simulink model "QCar2_Physical"  (R2025b)
settings: Solver=ode1  StartTime=0.0  StopTime=inf  FixedStep=Controller_Sample_Time  RelTol=1e-3  EnableMultiTasking=on
PreLoadFcn:
  | QCarSetup
values from neighbouring files (symbols this model uses):
  Audio_Sample_Time = 0.3    [QCarSetup.m]
  CSI_Sample_Time = 1/60    (= 0.0166666666667)    [QCarSetup.m]
  ImageDisplay_Sample_Time = 120*Controller_Sample_Time    (= 0.1)    [QCarSetup.m]
  LiDAR_Sample_Time = CSI_Sample_Time*3    (= 0.05)    [QCarSetup.m]
  NN_Sample_Time = RealSense_Sample_Time*1    (= 0.0333333333333)    [QCarSetup.m]
  RealSense_Sample_Time = CSI_Sample_Time*2    (= 0.0333333333333)    [QCarSetup.m]
undefined symbols (not defined in the file or in its folder): Cobra_Start, DiscIntNeverNeededParam, engine, gcbh, height, HIL, honk, Joystick_Sample_Time, JPEG, left, Point, put_me_down, qc_get_step_size, top, truck_start, video_display_show, width
libraries: quarc_library x55, simulink x4, simulink_extras x1, visiontextngfix x1
(part 2 of 3)

== system QCar2_Physical/QCar/QCar Control/powerConsumptionMonitor ==
  note: Battery percentage calculation
  note: P = VI
  note: Electrical
      | power
      | consumed
  note: Power Monitoring Module:
      |
      | This subsystem monitors power consumption and provides a percentage battery remaining indicator.
      |
      | Inputs:
      | motorCurrent (A) n/a : Motor current being pulled by the main drive motor
      | batteryVoltage (V) {0, 12.6} : Current battery voltage reading
      |
      | Outputs:
      | motorPowerConsumption (W) n/a : Current power in Watts being pulled by the main drive motor
      | batteryLevel (%) {0,1} : Percentage battery level remaining
      |
      | Usage:
      | This is based on a maximum 3S battery voltage of 12.6 V (4.2V per cell) and minimum of 10.5 V (3.5V per cell)
  motorCurrent (A) [1] : Inport
  batteryVoltage (V) [1] : Inport  Port=2
  Divide : Product  Inputs=*/
  Gain : Gain  Gain=100
  Product : Product
  Subtract : Sum  Inputs=+-
  Subtract1 : Sum  Inputs=+-
  max voltage : Constant  Value=12.6
  min voltage : Constant  Value=10.5
  motorPowerConsumption (W) [1] : Outport  VectorParamsAs1DForOutWhenUnconnected=off
  batteryLevel (%) [1] : Outport  Port=2  VectorParamsAs1DForOutWhenUnconnected=off
  wires:
  Divide/1 -> Gain/1
  Subtract1/1 -> Divide/2
  Gain/1 -> batteryLevel (%) [1]/1
  Product/1 -> motorPowerConsumption (W) [1]/1
  min voltage/1 -> Subtract/2, Subtract1/2
  motorCurrent (A) [1]/1 -> Product/1
  max voltage/1 -> Subtract1/1
  Subtract/1 -> Divide/1
  batteryVoltage (V) [1]/1 -> Subtract/1, Product/2

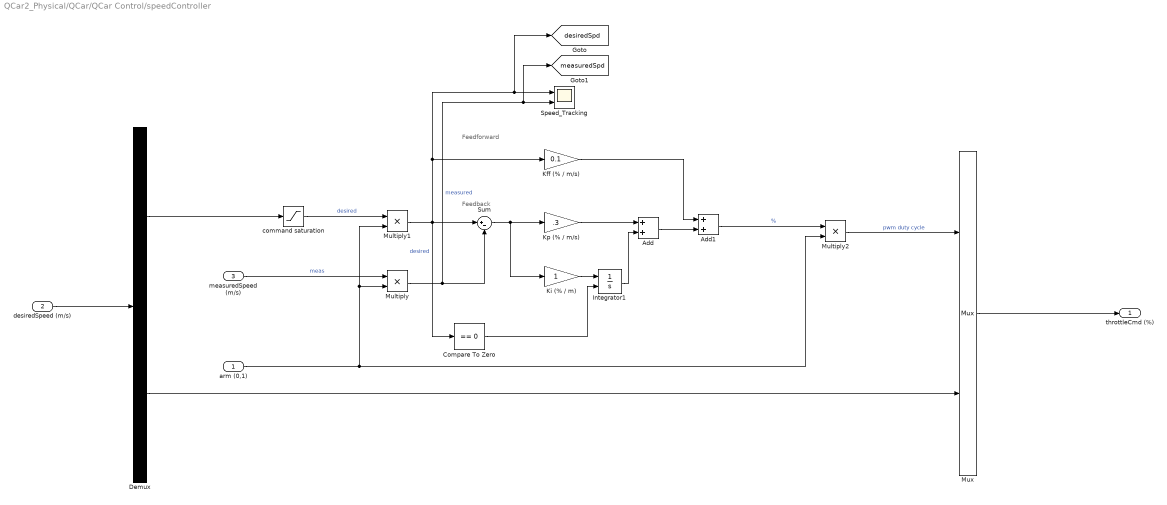
== system QCar2_Physical/QCar/QCar Control/speedController ==
  note: Feedforward
  note: Feedback
  arm (0,1) : Inport
  desiredSpeed (m/s) : Inport  Port=2
  measuredSpeed (m/s) : Inport  Port=3
  Add : Sum
  Add1 : Sum
  Compare To Zero : simulink/Logic and Bit Operations/Compare To Zero  relop===  OutDataTypeStr=boolean
  Demux : Demux  Outputs=2
  Integrator1 : Integrator  ExternalReset=either  LimitOutput=on  UpperSaturationLimit=0.4  LowerSaturationLimit=-0.4
  Kff (% / m/s) : Gain  Gain=0.1
  "Ki (% / m) " : Gain
  Kp (% / m/s) : Gain  Gain=.3
  Multiply : Product
  Multiply1 : Product
  Multiply2 : Product
  Mux : Mux  Inputs=2
  Speed_Tracking : Scope  NumInputPorts=2
      settings: TimeSpan=5  Title=Control Performance  ActiveDisplayYMinimum=-0.12863  ActiveDisplayYMaximum=1.15763  YLabel=m/s
  Sum : Sum  Inputs=|+-
  command saturation : Saturate  UpperLimit=5  LowerLimit=-5
  throttleCmd (%) : Outport  VectorParamsAs1DForOutWhenUnconnected=off
  tag scope: desiredSpd=global, measuredSpd=global
  wires:
  command saturation/1 -> Multiply1/1  "desired"
  arm (0,1)/1 -> Multiply1/2, Multiply/2, Multiply2/2
  measuredSpeed (m/s)/1 -> Multiply/1  "meas"
  Multiply/1 -> Sum/2, [measuredSpd], Speed_Tracking/2  "measured"
  Add/1 -> Add1/2
  Add1/1 -> Multiply2/1  "%"
  Multiply1/1 -> Compare To Zero/1, Sum/1, Kff (% / m/s)/1, [desiredSpd], Speed_Tracking/1  "desired"
  Integrator1/1 -> Add/2
  Kp (% / m/s)/1 -> Add/1
  Compare To Zero/1 -> Integrator1/2
  Kff (% / m/s)/1 -> Add1/1
  Sum/1 -> "Ki (% / m) "/1, Kp (% / m/s)/1
  "Ki (% / m) "/1 -> Integrator1/1
  Multiply2/1 -> Mux/1  "pwm duty cycle"
  Mux/1 -> throttleCmd (%)/1
  desiredSpeed (m/s)/1 -> Demux/1
  Demux/1 -> command saturation/1
  Demux/2 -> Mux/2

== system QCar2_Physical/QCar/QCar Control/turnSpeedHandling ==
  Commands in : Inport
  Cos ^ : Inport  Port=2
  Cos : Trigonometry  Operator=cos
  Demux1 : Demux  Outputs=2
  Mux : Mux  Inputs=2
  Product : Product
  Saturation : Saturate  UpperLimit=1  LowerLimit=.3
  Scope : Scope  NumInputPorts=2
      settings: Title=Turn-Speed Handling  ActiveDisplayYMinimum=-1  ActiveDisplayYMaximum=1  YLabel=m/s  DataLoggingVariableName=ScopeData2
  Scope1 : Scope  NumInputPorts=2
      settings: ActiveDisplayYMinimum=-0.6875  ActiveDisplayYMaximum=1.1875
  Square : Math  Operator=pow  SignedPower=on
  Commands : Outport  VectorParamsAs1DForOutWhenUnconnected=off
  wires:
  Cos/1 -> Square/1
  Saturation/1 -> Product/2
  Demux1/1 -> Product/1, Scope/1  "Speed Command"
  Commands in/1 -> Demux1/1
  Cos ^/1 -> Square/2
  Square/1 -> Saturation/1, Scope1/1
  Product/1 -> Mux/1, Scope/2
  Mux/1 -> Commands/1
  Demux1/2 -> Mux/2, Scope1/2, Cos/1

== system QCar2_Physical/RealSense Camera/Obstacle Detection/depth image processing ==
  imageDepth : Inport
  "Gain to increase \"brightness\"" : Gain  Gain=50
  Image Filter1 : quarc_library/Image Processing/Generic/Image Filter  filter_type=Depth hole-fill  source_of_roi=Internal dialog parameter  roi_style=[top, left, height, width]  roi=[]  maximum_roi=[]  roi_zone=Operate inside region of interest  border_type=Replicate  border_value=[0 0 0]  kernel_size=5  sigma=10  mask_size=[3 3]  kernel=int16([-2 -1 0; -1 1 1; 0 1 2])  divisor=1  offset=0  rounding=Nearest  algorithm_hint=None  threshold=100  alpha=0.9  num_frames=8  num_valid=1  gap_threshold=10  depth_threshold=255  iterations=2  norm_type=L1
      settings: AttributesFormatString=(%<filter_type>)  SourceProductName=QUARC Targets
  Image Filter2 : quarc_library/Image Processing/Generic/Image Filter  filter_type=Depth temporal low-pass  source_of_roi=Internal dialog parameter  roi_style=[top, left, height, width]  roi=[]  maximum_roi=[]  roi_zone=Operate inside region of interest  border_type=Replicate  border_value=[0 0 0]  kernel_size=5  sigma=10  mask_size=[3 3]  kernel=int16([-2 -1 0; -1 1 1; 0 1 2])  divisor=1  offset=0  rounding=Nearest  algorithm_hint=None  threshold=100  alpha=0.9  num_frames=8  num_valid=1  gap_threshold=10  depth_threshold=255  iterations=2  norm_type=L1
      settings: AttributesFormatString=(%<filter_type>)  SourceProductName=QUARC Targets
  Image Transform1 : quarc_library/Image Processing/Generic/Image Transform  algorithm=Colorize  color_theme=KRYGCBMW  min_pixel=0  max_pixel=255  contour_depth=1  focal_length=308  principal_point=[262 334]  radial_coeffs=[-0.3129 0.0907]  tangential_coeffs=[]  extrapolated_pixel=0  interpolation=nearest  row_coords=0  column_coords=0  output_height=480  output_width=640  angle=0  origin=[240 320]  output_origin=[240 320]  output_data_type=uint8
      settings: AttributesFormatString=(%<algorithm>)  SourceProductName=QUARC Targets
  Image Transform2 : quarc_library/Image Processing/Generic/Image Transform  algorithm=Decolorize  color_theme=KRYGCBMW  min_pixel=0  max_pixel=255  contour_depth=1  focal_length=308  principal_point=[262 334]  radial_coeffs=[-0.3129 0.0907]  tangential_coeffs=[]  extrapolated_pixel=0  interpolation=nearest  row_coords=0  column_coords=0  output_height=480  output_width=640  angle=0  origin=[240 320]  output_origin=[240 320]  output_data_type=uint8
      settings: AttributesFormatString=(%<algorithm>)  SourceProductName=QUARC Targets
  Manual Switch : ManualSwitch  CurrentSetting=0
  Manual Switch1 : ManualSwitch  CurrentSetting=0
  img_in : Outport
  wires:
  Image Filter2/1 -> Manual Switch/1
  Manual Switch/1 -> Image Filter1/1, Manual Switch1/2
  Image Filter1/1 -> Manual Switch1/1
  imageDepth/1 -> Image Filter2/1, Manual Switch/2
  Image Transform1/1 -> Image Transform2/1
  Image Transform2/1 -> img_in/1
  "Gain to increase \"brightness\""/1 -> Image Transform1/1
  Manual Switch1/1 -> "Gain to increase \"brightness\""/1

== system QCar2_Physical/RealSense Camera/RealSense Capture/Subsystem ==
  In1 : Inport
  Image Filter1 : quarc_library/Image Processing/Generic/Image Filter  filter_type=Depth hole-fill  source_of_roi=Internal dialog parameter  roi_style=[top, left, height, width]  roi=[]  maximum_roi=[]  roi_zone=Operate inside region of interest  border_type=Replicate  border_value=[0 0 0]  kernel_size=5  sigma=10  mask_size=[3 3]  kernel=int16([-2 -1 0; -1 1 1; 0 1 2])  divisor=1  offset=0  rounding=Nearest  algorithm_hint=None  threshold=100  alpha=0.9  num_frames=8  num_valid=1  gap_threshold=10  depth_threshold=255  iterations=2  norm_type=L1
      settings: AttributesFormatString=(%<filter_type>)  SourceProductName=QUARC Targets
  Image Filter2 : quarc_library/Image Processing/Generic/Image Filter  filter_type=Depth temporal low-pass  source_of_roi=Internal dialog parameter  roi_style=[top, left, height, width]  roi=[]  maximum_roi=[]  roi_zone=Operate inside region of interest  border_type=Replicate  border_value=[0 0 0]  kernel_size=5  sigma=10  mask_size=[3 3]  kernel=int16([-2 -1 0; -1 1 1; 0 1 2])  divisor=1  offset=0  rounding=Nearest  algorithm_hint=None  threshold=100  alpha=0.9  num_frames=8  num_valid=1  gap_threshold=10  depth_threshold=255  iterations=2  norm_type=L1
      settings: AttributesFormatString=(%<filter_type>)  SourceProductName=QUARC Targets
  Manual Switch : ManualSwitch
  Manual Switch1 : ManualSwitch
  Out1 : Outport
  wires:
  Image Filter1/1 -> Manual Switch1/1
  In1/1 -> Image Filter2/1, Manual Switch/2
  Manual Switch/1 -> Image Filter1/1, Manual Switch1/2
  Image Filter2/1 -> Manual Switch/1
  Manual Switch1/1 -> Out1/1

== system QCar2_Physical/RealSense Camera/RealSense Capture/yolo_stream ==
  depth : Inport
  rgb : Inport  Port=2
  new : Inport  Port=3
  AND : Logic  AllPortsSameDT=off  OutDataTypeStr=boolean
  AND1 : Logic  IconShape=distinctive  AllPortsSameDT=off  OutDataTypeStr=boolean
  Compare To Constant : simulink/Logic and Bit Operations/Compare To Constant  relop===  const=2  OutDataTypeStr=boolean
  Compare To Constant1 : simulink/Logic and Bit Operations/Compare To Constant  relop=>=  const=0  OutDataTypeStr=boolean
  Constant : Constant
  Constant1 : Constant
  Data Type Conversion : DataTypeConversion  OutDataTypeStr=fixdt('single', 'DataTypeOverride', 'Off')  SaturateOnIntegerOverflow=off  RndMeth=Floor
  Matrix Concatenate : Concatenate  Mode=Multidimensional array  ConcatenateDimension=3
  Memory : Memory  InheritSampleTime=on
  Stream Server : quarc_library/Communications/Basic/Stream Server  uri_source=Specify via dialog (do not evaluate)  uri=tcpip://remotehost:18777?nagle='on'  send_buffer_size=480*640*4*4  receive_buffer_size=480*640*3  byte_order=little endian (Intel - LSB first)  optimization=Minimum latency  send_options=Send most recent data  receive_options=Receive most recent data  default_value=uint8(zeros(480,640,3))  sample_time=qc_get_step_size*ceil(0.033 / qc_get_step_size)  active=off  implementation=Use blocking I/O in a separate thread  send_fifo_size=1000  receive_fifo_size=1000  send_priority=0  receive_priority=0  send_dimensions=off  receive_dimensions=off  max_dimensions=-1  data_type=uint8  type_expr=BusObject
      settings: AttributesFormatString="\"tcpip://remotehost:18777?nagle='on'\""
  Stream Server1 : quarc_library/Communications/Basic/Stream Server  uri_source=Specify via dialog (do not evaluate)  uri=tcpip://remotehost:18666?nagle='on'  send_buffer_size=4*2*4  receive_buffer_size=1440  byte_order=little endian (Intel - LSB first)  optimization=Minimum latency  send_options=Send most recent data  receive_options=Receive most recent data  default_value=zeros(4,2)  sample_time=qc_get_step_size*ceil(0.033 / qc_get_step_size)  active=off  implementation=Use blocking I/O in a separate thread  send_fifo_size=1000  receive_fifo_size=1000  send_priority=0  receive_priority=0  send_dimensions=off  receive_dimensions=off  max_dimensions=-1  data_type=single  type_expr=BusObject
      settings: AttributesFormatString="\"tcpip://remotehost:18666?nagle='on'\""
  Terminator3 : Terminator
  Terminator4 : Terminator
  Annotated Image : Outport
  Classification info : Outport  Port=2
  wires:
  Matrix Concatenate/1 -> Stream Server/1
  Stream Server/3 -> Terminator3/1
  Stream Server/5 -> Terminator4/1
  Data Type Conversion/1 -> Matrix Concatenate/2
  depth/1 -> Matrix Concatenate/1
  AND1/1 -> Stream Server/2
  rgb/1 -> Data Type Conversion/1
  Compare To Constant1/1 -> AND/2
  Stream Server/2 -> Compare To Constant1/1
  Stream Server/1 -> Compare To Constant/1
  Compare To Constant/1 -> AND/1
  AND/1 -> Memory/1
  new/1 -> AND1/1
  Memory/1 -> AND1/2
  Stream Server/4 -> Annotated Image/1
  Stream Server1/4 -> Classification info/1
  Constant/1 -> Stream Server1/2
  Constant1/1 -> Stream Server1/1

== system QCar2_Physical/VIsualization/LiDAR/captureLIDAR ==
  Display : Display
      settings: Decimation=100
  Display1 : Display
      settings: Decimation=100
  Display2 : Display
      settings: Decimation=100
  Ranging Sensor : quarc_library/Devices/Third-Party/Sensors/Ranging Sensor  sensor_type=RPLidar LIDAR  uri=serial-cpu://localhost:1?baud='256000',word='8',parity='none',stop='1',flow='none',dsr='on'  ranging_distance=Long  timing_budget=0.033  measurement_period=0.040  output_mode=Variable-size output  samples_per_revolution=1000  max_distance=0.050  max_angle=5  sample_time=LiDAR_Sample_Time  show_versions=on  active=on
      settings: SourceProductName=QUARC Targets
  distances (m) : Outport  VectorParamsAs1DForOutWhenUnconnected=off
  Heading (rad) : Outport  Port=2  VectorParamsAs1DForOutWhenUnconnected=off
  qual : Outport  Port=3  VectorParamsAs1DForOutWhenUnconnected=off
  new : Outport  Port=4  VectorParamsAs1DForOutWhenUnconnected=off
  wires:
  Ranging Sensor/1 -> distances (m)/1
  Ranging Sensor/3 -> Heading (rad)/1
  Ranging Sensor/4 -> qual/1
  Ranging Sensor/5 -> new/1
  Ranging Sensor/6 -> Display/1
  Ranging Sensor/7 -> Display1/1
  Ranging Sensor/8 -> Display2/1

== system QCar2_Physical/VIsualization/Rate Timing Plots/monitorTiming ==
  note: Timing Performance
  note: moniorTiming Module:
      |
      | This subsystem outputs the sample time and computation time of the model.
      |
      | Outputs:
      | sampleTime (s) n/a : Sample time (unfiltered and filtered) in seconds.
      | computationTime (s) n/a : Computation time (unfiltered and filtered) in seconds.
      |
      | Usage:
      | Compare the Sample Time (s) output to a constant (qc_get_step_size) to monitor whether or not the desired sample time is being achieved. The Computation Time (s) values should be lower than the corresponding sample time value to ensure that the solver has enough time per time step.
  Computation Time : quarc_library/Sources/Time/Computation Time  sample_time=CSI_Sample_Time  use_model=on  use_cpu_time=off
  Constant : Constant  Value=CSI_Sample_Time  SampleTime=-1
  Mux : Mux  Inputs=3
  Sample Time : quarc_library/Sources/Time/Sample Time  Priority=-99  sample_time=CSI_Sample_Time
  Timing (s) : Outport  VectorParamsAs1DForOutWhenUnconnected=off
  wires:
  Computation Time/1 -> Mux/3
  Mux/1 -> Timing (s)/1
  Sample Time/1 -> Mux/1
  Constant/1 -> Mux/2

== system QCar2_Physical/VIsualization/Rate Timing Plots/monitorTiming1 ==
  note: moniorTiming Module:
      |
      | This subsystem outputs the sample time and computation time of the model.
      |
      | Outputs:
      | sampleTime (s) n/a : Sample time (unfiltered and filtered) in seconds.
      | computationTime (s) n/a : Computation time (unfiltered and filtered) in seconds.
      |
      | Usage:
      | Compare the Sample Time (s) output to a constant (qc_get_step_size) to monitor whether or not the desired sample time is being achieved. The Computation Time (s) values should be lower than the corresponding sample time value to ensure that the solver has enough time per time step.
  note: Timing Performance
  Computation Time : quarc_library/Sources/Time/Computation Time  sample_time=qc_get_step_size  use_model=on  use_cpu_time=off
  Constant : Constant  Value=qc_get_step_size  SampleTime=-1
  Mux : Mux  Inputs=3
  Sample Time : quarc_library/Sources/Time/Sample Time  Priority=-99  sample_time=qc_get_step_size
  Timing (s) : Outport  VectorParamsAs1DForOutWhenUnconnected=off
  wires:
  Constant/1 -> Mux/2
  Sample Time/1 -> Mux/1
  Mux/1 -> Timing (s)/1
  Computation Time/1 -> Mux/3

== system QCar2_Physical/VIsualization/Rate Timing Plots/monitorTiming2 ==
  note: moniorTiming Module:
      |
      | This subsystem outputs the sample time and computation time of the model.
      |
      | Outputs:
      | sampleTime (s) n/a : Sample time (unfiltered and filtered) in seconds.
      | computationTime (s) n/a : Computation time (unfiltered and filtered) in seconds.
      |
      | Usage:
      | Compare the Sample Time (s) output to a constant (qc_get_step_size) to monitor whether or not the desired sample time is being achieved. The Computation Time (s) values should be lower than the corresponding sample time value to ensure that the solver has enough time per time step.
  note: Timing Performance
  Computation Time : quarc_library/Sources/Time/Computation Time  sample_time=RealSense_Sample_Time  use_model=on  use_cpu_time=off
  Constant : Constant  Value=RealSense_Sample_Time  SampleTime=-1
  Mux : Mux  Inputs=3
  Sample Time : quarc_library/Sources/Time/Sample Time  Priority=-99  sample_time=RealSense_Sample_Time
  Timing (s) : Outport  VectorParamsAs1DForOutWhenUnconnected=off
  wires:
  Constant/1 -> Mux/2
  Sample Time/1 -> Mux/1
  Mux/1 -> Timing (s)/1
  Computation Time/1 -> Mux/3

== system QCar2_Physical/VIsualization/Rate Timing Plots/monitorTiming3 ==
  note: Timing Performance
  note: moniorTiming Module:
      |
      | This subsystem outputs the sample time and computation time of the model.
      |
      | Outputs:
      | sampleTime (s) n/a : Sample time (unfiltered and filtered) in seconds.
      | computationTime (s) n/a : Computation time (unfiltered and filtered) in seconds.
      |
      | Usage:
      | Compare the Sample Time (s) output to a constant (qc_get_step_size) to monitor whether or not the desired sample time is being achieved. The Computation Time (s) values should be lower than the corresponding sample time value to ensure that the solver has enough time per time step.
  Computation Time : quarc_library/Sources/Time/Computation Time  sample_time=ImageDisplay_Sample_Time  use_model=on  use_cpu_time=off
  Constant : Constant  Value=ImageDisplay_Sample_Time  SampleTime=-1
  Mux : Mux  Inputs=3
  Sample Time : quarc_library/Sources/Time/Sample Time  Priority=-99  sample_time=ImageDisplay_Sample_Time
  Timing (s) : Outport  VectorParamsAs1DForOutWhenUnconnected=off
  wires:
  Computation Time/1 -> Mux/3
  Mux/1 -> Timing (s)/1
  Sample Time/1 -> Mux/1
  Constant/1 -> Mux/2

== system QCar2_Physical/VIsualization/Rate Timing Plots/monitorTiming4 ==
  note: Timing Performance
  note: moniorTiming Module:
      |
      | This subsystem outputs the sample time and computation time of the model.
      |
      | Outputs:
      | sampleTime (s) n/a : Sample time (unfiltered and filtered) in seconds.
      | computationTime (s) n/a : Computation time (unfiltered and filtered) in seconds.
      |
      | Usage:
      | Compare the Sample Time (s) output to a constant (qc_get_step_size) to monitor whether or not the desired sample time is being achieved. The Computation Time (s) values should be lower than the corresponding sample time value to ensure that the solver has enough time per time step.
  Computation Time : quarc_library/Sources/Time/Computation Time  sample_time=Joystick_Sample_Time  use_model=on  use_cpu_time=off
  Constant : Constant  Value=Joystick_Sample_Time  SampleTime=-1
  Mux : Mux  Inputs=3
  Sample Time : quarc_library/Sources/Time/Sample Time  Priority=-99  sample_time=Joystick_Sample_Time
  Timing (s) : Outport  VectorParamsAs1DForOutWhenUnconnected=off
  wires:
  Computation Time/1 -> Mux/3
  Mux/1 -> Timing (s)/1
  Sample Time/1 -> Mux/1
  Constant/1 -> Mux/2

== system QCar2_Physical/VIsualization/Rate Timing Plots/monitorTiming5 ==
  note: moniorTiming Module:
      |
      | This subsystem outputs the sample time and computation time of the model.
      |
      | Outputs:
      | sampleTime (s) n/a : Sample time (unfiltered and filtered) in seconds.
      | computationTime (s) n/a : Computation time (unfiltered and filtered) in seconds.
      |
      | Usage:
      | Compare the Sample Time (s) output to a constant (qc_get_step_size) to monitor whether or not the desired sample time is being achieved. The Computation Time (s) values should be lower than the corresponding sample time value to ensure that the solver has enough time per time step.
  note: Timing Performance
  Computation Time : quarc_library/Sources/Time/Computation Time  sample_time=LiDAR_Sample_Time  use_model=on  use_cpu_time=off
  Constant : Constant  Value=LiDAR_Sample_Time  SampleTime=-1
  Mux : Mux  Inputs=3
  Sample Time : quarc_library/Sources/Time/Sample Time  Priority=-99  sample_time=LiDAR_Sample_Time
  Timing (s) : Outport  VectorParamsAs1DForOutWhenUnconnected=off
  wires:
  Constant/1 -> Mux/2
  Sample Time/1 -> Mux/1
  Mux/1 -> Timing (s)/1
  Computation Time/1 -> Mux/3

== system QCar2_Physical/VIsualization/Rate Timing Plots/monitorTiming6 ==
  note: Timing Performance
  note: moniorTiming Module:
      |
      | This subsystem outputs the sample time and computation time of the model.
      |
      | Outputs:
      | sampleTime (s) n/a : Sample time (unfiltered and filtered) in seconds.
      | computationTime (s) n/a : Computation time (unfiltered and filtered) in seconds.
      |
      | Usage:
      | Compare the Sample Time (s) output to a constant (qc_get_step_size) to monitor whether or not the desired sample time is being achieved. The Computation Time (s) values should be lower than the corresponding sample time value to ensure that the solver has enough time per time step.
  Computation Time : quarc_library/Sources/Time/Computation Time  sample_time=NN_Sample_Time  use_model=on  use_cpu_time=off
  Constant : Constant  Value=NN_Sample_Time  SampleTime=-1
  Mux : Mux  Inputs=3
  Sample Time : quarc_library/Sources/Time/Sample Time  Priority=-99  sample_time=NN_Sample_Time
  Timing (s) : Outport  VectorParamsAs1DForOutWhenUnconnected=off
  wires:
  Computation Time/1 -> Mux/3
  Mux/1 -> Timing (s)/1
  Sample Time/1 -> Mux/1
  Constant/1 -> Mux/2

== system QCar2_Physical/VIsualization/Rate Timing Plots/monitorTiming7 ==
  note: Timing Performance
  note: moniorTiming Module:
      |
      | This subsystem outputs the sample time and computation time of the model.
      |
      | Outputs:
      | sampleTime (s) n/a : Sample time (unfiltered and filtered) in seconds.
      | computationTime (s) n/a : Computation time (unfiltered and filtered) in seconds.
      |
      | Usage:
      | Compare the Sample Time (s) output to a constant (qc_get_step_size) to monitor whether or not the desired sample time is being achieved. The Computation Time (s) values should be lower than the corresponding sample time value to ensure that the solver has enough time per time step.
  Computation Time : quarc_library/Sources/Time/Computation Time  sample_time=1  use_model=on  use_cpu_time=off
  Constant : Constant  SampleTime=-1
  Mux : Mux  Inputs=3
  Sample Time : quarc_library/Sources/Time/Sample Time  Priority=-99  sample_time=1
  Timing (s) : Outport  VectorParamsAs1DForOutWhenUnconnected=off
  wires:
  Computation Time/1 -> Mux/3
  Mux/1 -> Timing (s)/1
  Sample Time/1 -> Mux/1
  Constant/1 -> Mux/2

== system QCar2_Physical/VIsualization/Rate Timing Plots/monitorTiming8 ==
  note: moniorTiming Module:
      |
      | This subsystem outputs the sample time and computation time of the model.
      |
      | Outputs:
      | sampleTime (s) n/a : Sample time (unfiltered and filtered) in seconds.
      | computationTime (s) n/a : Computation time (unfiltered and filtered) in seconds.
      |
      | Usage:
      | Compare the Sample Time (s) output to a constant (qc_get_step_size) to monitor whether or not the desired sample time is being achieved. The Computation Time (s) values should be lower than the corresponding sample time value to ensure that the solver has enough time per time step.
  note: Timing Performance
  Computation Time : quarc_library/Sources/Time/Computation Time  sample_time=Audio_Sample_Time  use_model=on  use_cpu_time=off
  Constant : Constant  Value=Audio_Sample_Time  SampleTime=-1
  Mux : Mux  Inputs=3
  Sample Time : quarc_library/Sources/Time/Sample Time  Priority=-99  sample_time=Audio_Sample_Time
  Timing (s) : Outport  VectorParamsAs1DForOutWhenUnconnected=off
  wires:
  Constant/1 -> Mux/2
  Sample Time/1 -> Mux/1
  Mux/1 -> Timing (s)/1
  Computation Time/1 -> Mux/3

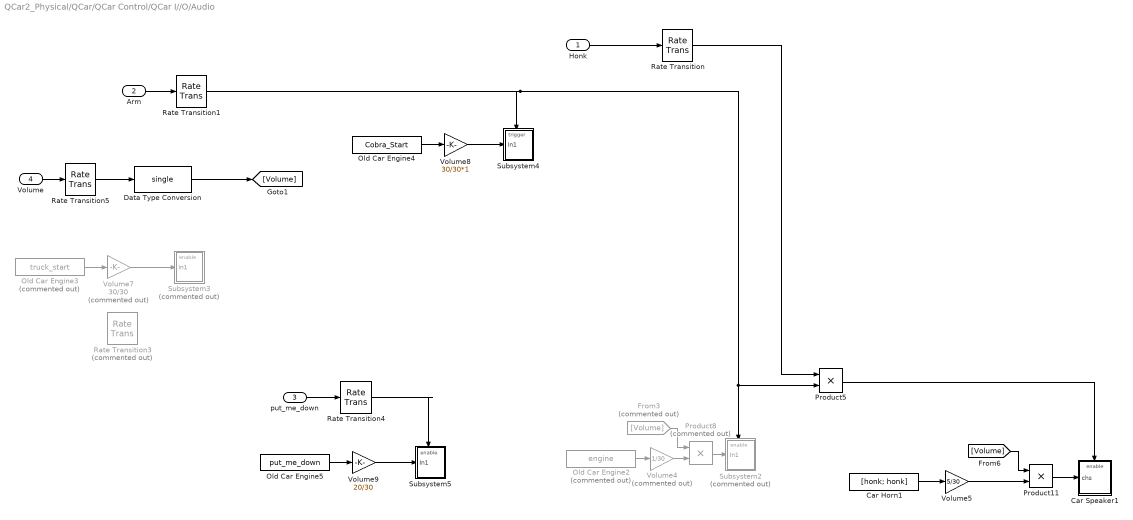
== system QCar2_Physical/QCar/QCar Control/QCar I//O/Audio ==
  Honk : Inport
  Arm : Inport  Port=2
  put_me_down : Inport  Port=3
  Volume : Inport  Port=4
  Car Horn1 : Constant  Value=[honk; honk]  VectorParams1D=off  OutDataTypeStr=single  SampleTime=Audio_Sample_Time
  Car Speaker1 : Subsystem
  Data Type Conversion : DataTypeConversion  OutDataTypeStr=single  SaturateOnIntegerOverflow=off  RndMeth=Floor
  From3 : From  Commented=on  GotoTag=Volume
  Old Car Engine2 : Constant  Commented=on  Value=engine  VectorParams1D=off  OutDataTypeStr=single  SampleTime=Audio_Sample_Time
  Old Car Engine3 : Constant  Commented=on  Value=truck_start  VectorParams1D=off  OutDataTypeStr=single  SampleTime=1
  Old Car Engine4 : Constant  Value=Cobra_Start  VectorParams1D=off  OutDataTypeStr=single  SampleTime=Audio_Sample_Time
  Old Car Engine5 : Constant  Value=put_me_down  VectorParams1D=off  OutDataTypeStr=single  SampleTime=Audio_Sample_Time
  Product11 : Product
  Product5 : Product
  Product8 : Product  Commented=on
  Rate Transition{,1,4..5} (4 alike) : RateTransition
  Rate Transition3 : RateTransition  Commented=on
  Subsystem2 : Subsystem  Commented=on
  Subsystem3 : Subsystem  Commented=on
  Subsystem4 : Subsystem
  Subsystem5 : Subsystem
  Volume4 : Gain  Commented=on  Gain=1/30  ParamDataTypeStr=double  OutDataTypeStr=single
  Volume5 : Gain  Gain=5/30  ParamDataTypeStr=double  OutDataTypeStr=single
  Volume7 : Gain  Commented=on  Gain=30/30  ParamDataTypeStr=double  OutDataTypeStr=single
  Volume8 : Gain  Gain=30/30*1  ParamDataTypeStr=double  OutDataTypeStr=single
  Volume9 : Gain  Gain=20/30  ParamDataTypeStr=double  OutDataTypeStr=single
  wires:
  Honk/1 -> Rate Transition/1
  Arm/1 -> Rate Transition1/1
  Rate Transition1/1 -> Subsystem2/Enable, Product5/2, Subsystem4/Trigger
  Old Car Engine2/1 -> Volume4/1
  Rate Transition/1 -> Product5/1
  Car Horn1/1 -> Volume5/1
  Old Car Engine3/1 -> Volume7/1
  Volume7/1 -> Subsystem3/1(In1)
  Product5/1 -> Car Speaker1/Enable
  Old Car Engine5/1 -> Volume9/1
  Volume9/1 -> Subsystem5/1(In1)
  Rate Transition4/1 -> Subsystem5/Enable
  put_me_down/1 -> Rate Transition4/1
  Volume/1 -> Rate Transition5/1
  Rate Transition5/1 -> Data Type Conversion/1
  From3/1 -> Product8/1
  Product8/1 -> Subsystem2/1(In1)
  Volume4/1 -> Product8/2
  [Volume] -> Product11/1
  Product11/1 -> Car Speaker1/1(chs)
  Volume5/1 -> Product11/2
  Data Type Conversion/1 -> [Volume]
  Old Car Engine4/1 -> Volume8/1
  Volume8/1 -> Subsystem4/1(In1)

== system QCar2_Physical/QCar/QCar Control/QCar I//O/Greater Than Threshold ==
  Signal : Inport
  Threshold : Inport  Port=2
  Duration : Inport  Port=3
  Data Type Conversion : DataTypeConversion  SaturateOnIntegerOverflow=off  RndMeth=Floor
  Discrete-Time Integrator : DiscreteIntegrator  Priority=1  ExternalReset=level  SampleTime=qc_get_step_size  ICPrevOutput=DiscIntNeverNeededParam  ICPrevScaledInput=DiscIntNeverNeededParam
  Logical Operator : Logic  Operator=NOT  AllPortsSameDT=off  OutDataTypeStr=boolean
  Relational Operator : RelationalOperator  InputSameDT=off
  Relational Operator1 : RelationalOperator  InputSameDT=off
  elapsed : Outport  VectorParamsAs1DForOutWhenUnconnected=off
  time : Outport  Port=2  VectorParamsAs1DForOutWhenUnconnected=off
  wires:
  Relational Operator1/1 -> elapsed/1
  Duration/1 -> Relational Operator1/2
  Discrete-Time Integrator/1 -> time/1, Relational Operator1/1
  Logical Operator/1 -> Discrete-Time Integrator/2
  Relational Operator/1 -> Logical Operator/1, Data Type Conversion/1
  Threshold/1 -> Relational Operator/2
  Signal/1 -> Relational Operator/1
  Data Type Conversion/1 -> Discrete-Time Integrator/1

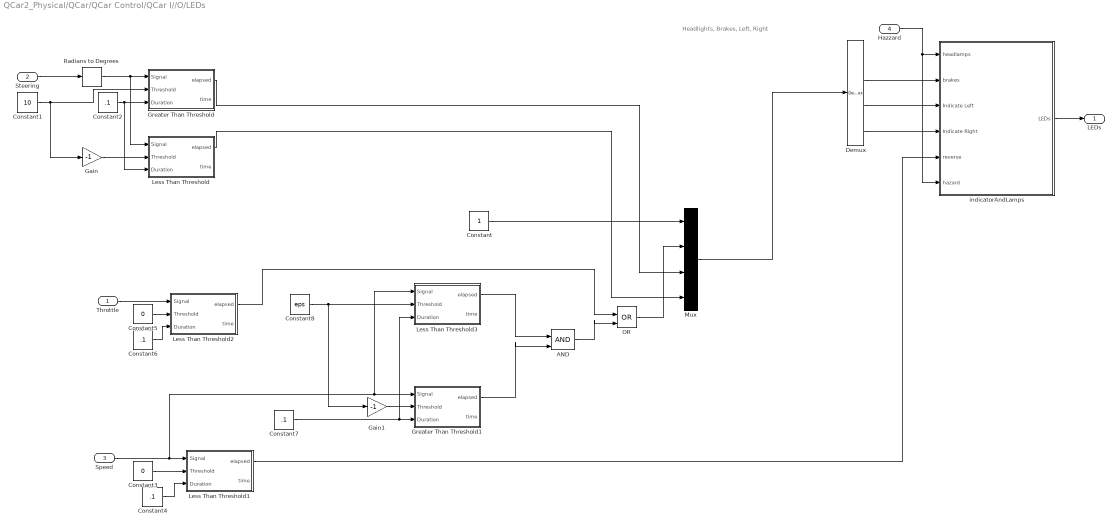
== system QCar2_Physical/QCar/QCar Control/QCar I//O/LEDs ==
  note: Headlights, Brakes, Left, Right
  Throttle : Inport
  Steering : Inport  Port=2
  Speed : Inport  Port=3
  Hazzard : Inport  Port=4
  AND : Logic  IconShape=distinctive  AllPortsSameDT=off  OutDataTypeStr=boolean
  Constant : Constant  OutDataTypeStr=boolean
  Constant1 : Constant  Value=10
  Constant{2,4,6..7} (4 alike) : Constant  Value=.1
  Constant3 : Constant  Value=0
  Constant5 : Constant  Value=0
  Constant8 : Constant  Value=eps
  Demux : Demux
  Gain : Gain  Gain=-1
  Gain1 : Gain  Gain=-1
  Greater Than Threshold : Subsystem
  Greater Than Threshold1 : Subsystem
  Less Than Threshold : Subsystem
  Less Than Threshold1 : Subsystem
  Less Than Threshold2 : Subsystem
  Less Than Threshold3 : Subsystem
  Mux : Mux
  OR : Logic  Operator=OR  IconShape=distinctive  AllPortsSameDT=off  OutDataTypeStr=boolean
  Radians to Degrees : simulink_extras/Transformations/Radians to Degrees
  indicatorAndLamps : Subsystem
  LEDs : Outport
  wires:
  indicatorAndLamps/1(LEDs) -> LEDs/1
  Steering/1 -> Radians to Degrees/1
  Radians to Degrees/1 -> Less Than Threshold/1(Signal), Greater Than Threshold/1(Signal)
  Constant1/1 -> Gain/1, Greater Than Threshold/2(Threshold)
  Constant2/1 -> Less Than Threshold/3(Duration), Greater Than Threshold/3(Duration)
  Greater Than Threshold/1(elapsed) -> Mux/3
  Gain/1 -> Less Than Threshold/2(Threshold)
  Less Than Threshold/1(elapsed) -> Mux/4
  Speed/1 -> Less Than Threshold3/1(Signal), Greater Than Threshold1/1(Signal), Less Than Threshold1/1(Signal)
  Constant3/1 -> Less Than Threshold1/2(Threshold)
  Constant4/1 -> Less Than Threshold1/3(Duration)
  Less Than Threshold1/1(elapsed) -> indicatorAndLamps/5(reverse)
  Throttle/1 -> Less Than Threshold2/1(Signal)
  Constant5/1 -> Less Than Threshold2/2(Threshold)
  Constant6/1 -> Less Than Threshold2/3(Duration)
  Hazzard/1 -> indicatorAndLamps/6(hazard), indicatorAndLamps/1(headlamps)
  Less Than Threshold2/1(elapsed) -> OR/1
  Constant7/1 -> Less Than Threshold3/3(Duration), Greater Than Threshold1/3(Duration)
  Constant8/1 -> Gain1/1, Less Than Threshold3/2(Threshold)
  Less Than Threshold3/1(elapsed) -> AND/1
  Greater Than Threshold1/1(elapsed) -> AND/2
  AND/1 -> OR/2
  Gain1/1 -> Greater Than Threshold1/2(Threshold)
  Constant/1 -> Mux/1
  OR/1 -> Mux/2
  Demux/3 -> indicatorAndLamps/3(Indicate Left)
  Demux/2 -> indicatorAndLamps/2(brakes)
  Demux/4 -> indicatorAndLamps/4(Indicate Right)
  Mux/1 -> Demux/1

== system QCar2_Physical/QCar/QCar Control/QCar I//O/Less Than Threshold1 ==
  Signal : Inport
  Threshold : Inport  Port=2
  Duration : Inport  Port=3
  Data Type Conversion : DataTypeConversion  SaturateOnIntegerOverflow=off  RndMeth=Floor
  Discrete-Time Integrator : DiscreteIntegrator  Priority=1  ExternalReset=level  SampleTime=qc_get_step_size  ICPrevOutput=DiscIntNeverNeededParam  ICPrevScaledInput=DiscIntNeverNeededParam
  Logical Operator : Logic  Operator=NOT  AllPortsSameDT=off  OutDataTypeStr=boolean
  Relational Operator : RelationalOperator  Operator=<  InputSameDT=off
  Relational Operator1 : RelationalOperator  InputSameDT=off
  elapsed : Outport  VectorParamsAs1DForOutWhenUnconnected=off
  time : Outport  Port=2  VectorParamsAs1DForOutWhenUnconnected=off
  wires:
  Data Type Conversion/1 -> Discrete-Time Integrator/1
  Signal/1 -> Relational Operator/1
  Threshold/1 -> Relational Operator/2
  Relational Operator/1 -> Data Type Conversion/1, Logical Operator/1
  Logical Operator/1 -> Discrete-Time Integrator/2
  Discrete-Time Integrator/1 -> Relational Operator1/1, time/1
  Duration/1 -> Relational Operator1/2
  Relational Operator1/1 -> elapsed/1

== system QCar2_Physical/QCar/QCar Control/QCar I//O/basicSpeedEstimation ==
  note: speedEstimation Module:
      |
      | This subsystem converts the motor speed measurements in counts/s to a useful longitudinal car speed in m/s.
      |
      | Inputs:
      | motorSpeed (counts/s) n/a : Drive motor speed measured using an encoder
      |
      | Outputs:
      | longitudinalCarSpeed (m/s) n/a : The platform's longitudinal speed (along the front-rear axis direction)
  note: (Diff. pinion*pinion)/(Spur*Diff. spur)
  note: v = 2*pi*r * omega (if omega is in rot/s)
      | v = r * omega (if omega is in rad/s)
      | r = 0.0342 m
  note: Estimate car speed from motor encoder counts rate
  motorSpeed (counts/s) : Inport
  counts to rotations : Gain  Gain=1/720/4
  gear ratios : Gain  Gain=(13*19)/(70*37)
  rot/s to rad/s : Gain  Gain=2*pi
  wheel radius : Gain  Gain=0.0342
  longitudinalCarSpeed (m/s) : Outport  VectorParamsAs1DForOutWhenUnconnected=off
  wires:
  gear ratios/1 -> rot/s to rad/s/1  "shaft speed (rots/s)"
  wheel radius/1 -> longitudinalCarSpeed (m/s)/1  "wheel speed (m/s)"
  counts to rotations/1 -> gear ratios/1  "motor speed (rot/s)"
  rot/s to rad/s/1 -> wheel radius/1  "wheel speed (rad/s)"
  motorSpeed (counts/s)/1 -> counts to rotations/1

== system QCar2_Physical/QCar/QCar Control/QCar I//O/basicSpeedEstimation1 ==
  note: Estimate car speed from motor encoder counts rate
  note: v = 2*pi*r * omega (if omega is in rot/s)
      | v = r * omega (if omega is in rad/s)
      | r = 0.0342 m
  note: (Diff. pinion*pinion)/(Spur*Diff. spur)
  note: speedEstimation Module:
      |
      | This subsystem converts the motor speed measurements in counts/s to a useful longitudinal car speed in m/s.
      |
      | Inputs:
      | motorSpeed (counts/s) n/a : Drive motor speed measured using an encoder
      |
      | Outputs:
      | longitudinalCarSpeed (m/s) n/a : The platform's longitudinal speed (along the front-rear axis direction)
  motorSpeed (counts/s) : Inport
  counts to rotations : Gain  Gain=1/720/4
  gear ratios : Gain  Gain=(13*19)/(70*37)
  rot/s to rad/s : Gain  Gain=2*pi
  wheel radius : Gain  Gain=0.0342
  longitudinalCarSpeed (m/s) : Outport  VectorParamsAs1DForOutWhenUnconnected=off
  wires:
  motorSpeed (counts/s)/1 -> counts to rotations/1
  rot/s to rad/s/1 -> wheel radius/1  "wheel speed (rad/s)"
  counts to rotations/1 -> gear ratios/1  "motor speed (rot/s)"
  wheel radius/1 -> longitudinalCarSpeed (m/s)/1  "wheel speed (m/s)"
  gear ratios/1 -> rot/s to rad/s/1  "shaft speed (rots/s)"

== system QCar2_Physical/QCar/QCar Control/QCar I//O/Audio/Car Speaker1 ==
  chs : Inport
  Enable : EnablePort
  Audio Play : quarc_library/Multimedia/Audio Play  device_id=demixer  sample_rate=44100  num_channels=[]  buffer_size=44100  sample_time=-1
      settings: SourceProductName=QUARC Targets
  wires:
  chs/1 -> Audio Play/1

== system QCar2_Physical/QCar/QCar Control/QCar I//O/Audio/Subsystem2 ==
  In1 : Inport
  Enable : EnablePort
  Audio Play : quarc_library/Multimedia/Audio Play  device_id=demixer  sample_rate=41000  num_channels=[]  buffer_size=length (engine)  sample_time=-1
      settings: SourceProductName=QUARC Targets
  wires:
  In1/1 -> Audio Play/1

== system QCar2_Physical/QCar/QCar Control/QCar I//O/Audio/Subsystem3 ==
  In1 : Inport
  Enable : EnablePort
  Audio Play : quarc_library/Multimedia/Audio Play  device_id=demixer  sample_rate=48000  num_channels=[]  buffer_size=length(truck_start)  sample_time=-1
      settings: SourceProductName=QUARC Targets
  wires:
  In1/1 -> Audio Play/1

== system QCar2_Physical/QCar/QCar Control/QCar I//O/Audio/Subsystem4 ==
  In1 : Inport
  Trigger : TriggerPort  VariantControl=Variant  PortDimensions=1
  Audio Play : quarc_library/Multimedia/Audio Play  device_id=demixer  sample_rate=48000  num_channels=[]  buffer_size=length(Cobra_Start)  sample_time=-1
      settings: SourceProductName=QUARC Targets
  wires:
  In1/1 -> Audio Play/1

== system QCar2_Physical/QCar/QCar Control/QCar I//O/Audio/Subsystem5 ==
  In1 : Inport
  Enable : EnablePort
  Audio Play : quarc_library/Multimedia/Audio Play  device_id=demixer  sample_rate=48000  num_channels=[]  buffer_size=length(put_me_down)  sample_time=-1
      settings: SourceProductName=QUARC Targets
  wires:
  In1/1 -> Audio Play/1

== system QCar2_Physical/QCar/QCar Control/QCar I//O/LEDs/Greater Than Threshold ==
  Signal : Inport
  Threshold : Inport  Port=2
  Duration : Inport  Port=3
  Data Type Conversion : DataTypeConversion  SaturateOnIntegerOverflow=off  RndMeth=Floor
  Discrete-Time Integrator : DiscreteIntegrator  Priority=1  ExternalReset=level  SampleTime=qc_get_step_size  ICPrevOutput=DiscIntNeverNeededParam  ICPrevScaledInput=DiscIntNeverNeededParam
  Logical Operator : Logic  Operator=NOT  AllPortsSameDT=off  OutDataTypeStr=boolean
  Relational Operator : RelationalOperator  InputSameDT=off
  Relational Operator1 : RelationalOperator  InputSameDT=off
  elapsed : Outport  VectorParamsAs1DForOutWhenUnconnected=off
  time : Outport  Port=2  VectorParamsAs1DForOutWhenUnconnected=off
  wires:
  Relational Operator1/1 -> elapsed/1
  Duration/1 -> Relational Operator1/2
  Discrete-Time Integrator/1 -> time/1, Relational Operator1/1
  Logical Operator/1 -> Discrete-Time Integrator/2
  Relational Operator/1 -> Logical Operator/1, Data Type Conversion/1
  Threshold/1 -> Relational Operator/2
  Signal/1 -> Relational Operator/1
  Data Type Conversion/1 -> Discrete-Time Integrator/1

== system QCar2_Physical/QCar/QCar Control/QCar I//O/LEDs/Greater Than Threshold1 ==
  Signal : Inport
  Threshold : Inport  Port=2
  Duration : Inport  Port=3
  Data Type Conversion : DataTypeConversion  SaturateOnIntegerOverflow=off  RndMeth=Floor
  Discrete-Time Integrator : DiscreteIntegrator  Priority=1  ExternalReset=level  SampleTime=qc_get_step_size  ICPrevOutput=DiscIntNeverNeededParam  ICPrevScaledInput=DiscIntNeverNeededParam
  Logical Operator : Logic  Operator=NOT  AllPortsSameDT=off  OutDataTypeStr=boolean
  Relational Operator : RelationalOperator  InputSameDT=off
  Relational Operator1 : RelationalOperator  InputSameDT=off
  elapsed : Outport  VectorParamsAs1DForOutWhenUnconnected=off
  time : Outport  Port=2  VectorParamsAs1DForOutWhenUnconnected=off
  wires:
  Relational Operator1/1 -> elapsed/1
  Duration/1 -> Relational Operator1/2
  Discrete-Time Integrator/1 -> time/1, Relational Operator1/1
  Logical Operator/1 -> Discrete-Time Integrator/2
  Relational Operator/1 -> Logical Operator/1, Data Type Conversion/1
  Threshold/1 -> Relational Operator/2
  Signal/1 -> Relational Operator/1
  Data Type Conversion/1 -> Discrete-Time Integrator/1

== system QCar2_Physical/QCar/QCar Control/QCar I//O/LEDs/Less Than Threshold ==
  Signal : Inport
  Threshold : Inport  Port=2
  Duration : Inport  Port=3
  Data Type Conversion : DataTypeConversion  SaturateOnIntegerOverflow=off  RndMeth=Floor
  Discrete-Time Integrator : DiscreteIntegrator  Priority=1  ExternalReset=level  SampleTime=qc_get_step_size  ICPrevOutput=DiscIntNeverNeededParam  ICPrevScaledInput=DiscIntNeverNeededParam
  Logical Operator : Logic  Operator=NOT  AllPortsSameDT=off  OutDataTypeStr=boolean
  Relational Operator : RelationalOperator  Operator=<  InputSameDT=off
  Relational Operator1 : RelationalOperator  InputSameDT=off
  elapsed : Outport  VectorParamsAs1DForOutWhenUnconnected=off
  time : Outport  Port=2  VectorParamsAs1DForOutWhenUnconnected=off
  wires:
  Relational Operator1/1 -> elapsed/1
  Duration/1 -> Relational Operator1/2
  Discrete-Time Integrator/1 -> time/1, Relational Operator1/1
  Logical Operator/1 -> Discrete-Time Integrator/2
  Relational Operator/1 -> Logical Operator/1, Data Type Conversion/1
  Threshold/1 -> Relational Operator/2
  Signal/1 -> Relational Operator/1
  Data Type Conversion/1 -> Discrete-Time Integrator/1

== system QCar2_Physical/QCar/QCar Control/QCar I//O/LEDs/Less Than Threshold1 ==
  Signal : Inport
  Threshold : Inport  Port=2
  Duration : Inport  Port=3
  Data Type Conversion : DataTypeConversion  SaturateOnIntegerOverflow=off  RndMeth=Floor
  Discrete-Time Integrator : DiscreteIntegrator  Priority=1  ExternalReset=level  SampleTime=qc_get_step_size  ICPrevOutput=DiscIntNeverNeededParam  ICPrevScaledInput=DiscIntNeverNeededParam
  Logical Operator : Logic  Operator=NOT  AllPortsSameDT=off  OutDataTypeStr=boolean
  Relational Operator : RelationalOperator  Operator=<  InputSameDT=off
  Relational Operator1 : RelationalOperator  InputSameDT=off
  elapsed : Outport  VectorParamsAs1DForOutWhenUnconnected=off
  time : Outport  Port=2  VectorParamsAs1DForOutWhenUnconnected=off
  wires:
  Data Type Conversion/1 -> Discrete-Time Integrator/1
  Signal/1 -> Relational Operator/1
  Threshold/1 -> Relational Operator/2
  Relational Operator/1 -> Data Type Conversion/1, Logical Operator/1
  Logical Operator/1 -> Discrete-Time Integrator/2
  Discrete-Time Integrator/1 -> Relational Operator1/1, time/1
  Duration/1 -> Relational Operator1/2
  Relational Operator1/1 -> elapsed/1

== system QCar2_Physical/QCar/QCar Control/QCar I//O/LEDs/Less Than Threshold2 ==
  Signal : Inport
  Threshold : Inport  Port=2
  Duration : Inport  Port=3
  Data Type Conversion : DataTypeConversion  SaturateOnIntegerOverflow=off  RndMeth=Floor
  Discrete-Time Integrator : DiscreteIntegrator  Priority=1  ExternalReset=level  SampleTime=qc_get_step_size  ICPrevOutput=DiscIntNeverNeededParam  ICPrevScaledInput=DiscIntNeverNeededParam
  Logical Operator : Logic  Operator=NOT  AllPortsSameDT=off  OutDataTypeStr=boolean
  Relational Operator : RelationalOperator  Operator=<  InputSameDT=off
  Relational Operator1 : RelationalOperator  InputSameDT=off
  elapsed : Outport  VectorParamsAs1DForOutWhenUnconnected=off
  time : Outport  Port=2  VectorParamsAs1DForOutWhenUnconnected=off
  wires:
  Relational Operator1/1 -> elapsed/1
  Duration/1 -> Relational Operator1/2
  Discrete-Time Integrator/1 -> time/1, Relational Operator1/1
  Logical Operator/1 -> Discrete-Time Integrator/2
  Relational Operator/1 -> Logical Operator/1, Data Type Conversion/1
  Threshold/1 -> Relational Operator/2
  Signal/1 -> Relational Operator/1
  Data Type Conversion/1 -> Discrete-Time Integrator/1

== system QCar2_Physical/QCar/QCar Control/QCar I//O/LEDs/Less Than Threshold3 ==
  Signal : Inport
  Threshold : Inport  Port=2
  Duration : Inport  Port=3
  Data Type Conversion : DataTypeConversion  SaturateOnIntegerOverflow=off  RndMeth=Floor
  Discrete-Time Integrator : DiscreteIntegrator  Priority=1  ExternalReset=level  SampleTime=qc_get_step_size  ICPrevOutput=DiscIntNeverNeededParam  ICPrevScaledInput=DiscIntNeverNeededParam
  Logical Operator : Logic  Operator=NOT  AllPortsSameDT=off  OutDataTypeStr=boolean
  Relational Operator : RelationalOperator  Operator=<  InputSameDT=off
  Relational Operator1 : RelationalOperator  InputSameDT=off
  elapsed : Outport  VectorParamsAs1DForOutWhenUnconnected=off
  time : Outport  Port=2  VectorParamsAs1DForOutWhenUnconnected=off
  wires:
  Data Type Conversion/1 -> Discrete-Time Integrator/1
  Signal/1 -> Relational Operator/1
  Threshold/1 -> Relational Operator/2
  Relational Operator/1 -> Data Type Conversion/1, Logical Operator/1
  Logical Operator/1 -> Discrete-Time Integrator/2
  Discrete-Time Integrator/1 -> Relational Operator1/1, time/1
  Duration/1 -> Relational Operator1/2
  Relational Operator1/1 -> elapsed/1

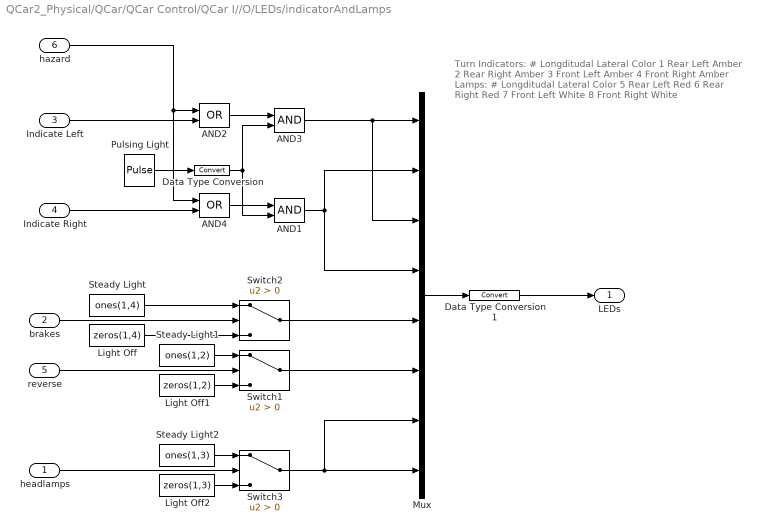
== system QCar2_Physical/QCar/QCar Control/QCar I//O/LEDs/indicatorAndLamps ==
  note: Turn Indicators:
      | # Longditudal Lateral Color
      | 1 Rear Left Amber
      | 2 Rear Right Amber
      | 3 Front Left Amber
      | 4 Front Right Amber
      |
      | Lamps:
      | # Longditudal Lateral Color
      | 5 Rear Left Red
      | 6 Rear Right Red
      | 7 Front Left White
      | 8 Front Right White
  headlamps : Inport
  brakes : Inport  Port=2
  Indicate Left : Inport  Port=3
  Indicate Right : Inport  Port=4
  reverse : Inport  Port=5
  hazard : Inport  Port=6
  AND1 : Logic  IconShape=distinctive  AllPortsSameDT=off  OutDataTypeStr=boolean
  AND2 : Logic  Operator=OR  IconShape=distinctive  AllPortsSameDT=off  OutDataTypeStr=boolean
  AND3 : Logic  IconShape=distinctive  AllPortsSameDT=off  OutDataTypeStr=boolean
  AND4 : Logic  Operator=OR  IconShape=distinctive  AllPortsSameDT=off  OutDataTypeStr=boolean
  Data Type Conversion : DataTypeConversion  SaturateOnIntegerOverflow=off  RndMeth=Floor
  Data Type Conversion1 : DataTypeConversion  SaturateOnIntegerOverflow=off  RndMeth=Floor
  Light Off : Constant  Value=zeros(1,4)  OutDataTypeStr=boolean
  Light Off1 : Constant  Value=zeros(1,2)  OutDataTypeStr=boolean
  Light Off2 : Constant  Value=zeros(1,3)  OutDataTypeStr=boolean
  Mux : Mux  Inputs=8
  Pulsing Light : DiscretePulseGenerator  Period=1/qc_get_step_size  PulseWidth=1/2/qc_get_step_size  SampleTime=qc_get_step_size
  Steady Light : Constant  Value=ones(1,4)  OutDataTypeStr=boolean
  Steady Light1 : Constant  Value=ones(1,2)  OutDataTypeStr=boolean
  Steady Light2 : Constant  Value=ones(1,3)  OutDataTypeStr=boolean
  Switch1 : Switch  Criteria=u2 > Threshold  SaturateOnIntegerOverflow=off  InputSameDT=off
  Switch2 : Switch  Criteria=u2 > Threshold  SaturateOnIntegerOverflow=off  InputSameDT=off
  Switch3 : Switch  Criteria=u2 > Threshold  SaturateOnIntegerOverflow=off  InputSameDT=off
  LEDs : Outport  VectorParamsAs1DForOutWhenUnconnected=off
  wires:
  Light Off/1 -> Switch2/3
  Steady Light/1 -> Switch2/1
  Indicate Right/1 -> AND4/2
  Mux/1 -> Data Type Conversion1/1
  Pulsing Light/1 -> Data Type Conversion/1
  Data Type Conversion/1 -> AND3/2, AND1/2
  Data Type Conversion1/1 -> LEDs/1
  Indicate Left/1 -> AND2/2
  Switch2/1 -> Mux/5
  AND3/1 -> Mux/3, Mux/1
  AND1/1 -> Mux/4, Mux/2
  Switch1/1 -> Mux/6
  Switch3/1 -> Mux/7, Mux/8
  brakes/1 -> Switch2/2
  reverse/1 -> Switch1/2
  headlamps/1 -> Switch3/2
  hazard/1 -> AND2/1, AND4/1
  AND2/1 -> AND3/1
  AND4/1 -> AND1/1
  Light Off1/1 -> Switch1/3
  Light Off2/1 -> Switch3/3
  Steady Light1/1 -> Switch1/1
  Steady Light2/1 -> Switch3/1

== matlab function QCar2_Physical/VIsualization/MATLAB Function1 ==
  settings: updateMethod=DISCRETE
  data: desired_speed input; speed_cmd output; desired_steering input; steering_cmd output; min_front input; min_left input; min_right input; dt input
function [speed_cmd, steering_cmd] = LiDAR_Avoidance_FSM(desired_speed, desired_steering, min_front, min_left, min_right, dt)
    % persistent variables สำหรับจำสถานะ FSM ใน Simulink
    persistent fsm_state avoid_dir
    if isempty(fsm_state)
        fsm_state = 0;   % 0: NORMAL DEMO, 1: AVOID_LEFT, 2: PASS, 3: RETURN
        avoid_dir = 1;   % 1: Left, -1: Right
    end

    % ค่าเริ่มต้นสำหรับ MATLAB Coder (ป้องกัน undefined execution paths)
    speed_cmd = desired_speed;
    steering_cmd = desired_steering;
    steer_angle = 0.42; % มุมพวงมาลัยหักหลบ (rad) (~24 องศา)

    switch fsm_state
        case 0 % NORMAL DEMO / LANE KEEPING (วิ่งตามเส้นทาง Demo ปกติ)
            speed_cmd = desired_speed;
            steering_cmd = desired_steering;
            % ตรวจจับสิ่งกีดขวางด้านหน้าในระยะ < 0.4m
            if min_front < 0.4
                fsm_state = 1; % เริ่มเบี่ยงออกทันที
                if min_left > 0.3 || min_left >= min_right
                    avoid_dir = -1;  % เบี่ยงซ้าย
                else
                    avoid_dir = 1; % เบี่ยงขวา
                end
            end

        case 1 % AVOIDING (หักเลี้ยวเบี่ยงออก)
            speed_cmd = 0.40;
            steering_cmd = -avoid_dir * steer_angle; % หักพวงมาลัยหลบออก
            if min_front < 0.4 && min_right < 0.3
                steering_cmd = avoid_dir * steer_angle;
            elseif min_front > 0.4
                fsm_state = 2; % เปลี่ยนเป็นแซง
            end

        case 2 % PASSING (ขับแซงขนาน)
            speed_cmd = 0.42;
            steering_cmd = desired_steering * 0.5; % ขับตามแนวเลนเดิมประคอง
            % เช็คว่าด้านข้าง (ฝั่งตรงข้ามกับที่เบี่ยงออก) โล่งพอที่จะกลับเข้าเลนได้
            if avoid_dir == -1
                side_clear = min_right; % เบี่ยงซ้ายไป ต้องเช็คขวาก่อนกลับเข้าเลน
            else
                side_clear = min_left;  % เบี่ยงขวาไป ต้องเช็คซ้ายก่อนกลับเข้าเลน
            end
            if side_clear > 0.3
                fsm_state = 3; % เปลี่ยนเป็นหักกลับเข้าเลน
            end

        case 3 % RETURNING (หักกลับเข้าเลนเดิม)
            speed_cmd = 0.40;
            steering_cmd = avoid_dir * steer_angle; % หักพวงมาลัยกลับเข้าเลน
            % เช็คว่ากลับเข้าเลนแล้ว: ด้านหน้าโล่ง และไม่มีอะไรใกล้ด้านข้างที่เบี่ยงออกไปแล้ว
            if avoid_dir == -1
                returned_clear = min_left; % เบี่ยงซ้ายไป เช็คซ้ายตอนจะกลับ
            else
                returned_clear = min_right;
            end
            if min_front > 0.4 && returned_clear > 0.3
                fsm_state = 0; % กลับเข้าโหมดวิ่งตาม Demo ปกติ
            end

        otherwise
            speed_cmd = desired_speed;
            steering_cmd = desired_steering;
            fsm_state = 0;
    end
end

== matlab function QCar2_Physical/VIsualization/MATLAB Function ==
  data: Distances input; min_front output; Headings input; min_left output; min_right output
function [min_front, min_left, min_right] = LiDAR_Obstacle_Detector(Distances, Headings)
    % แปลงมุม Headings (0..2*pi) ให้เป็นช่วง [-pi, pi]
    angles = atan2(sin(Headings), cos(Headings));
    
    % กรองระยะ: ต้องมากกว่า 0.15m (ตัดสัญญาณรบกวนโครงรถ) และน้อยกว่า 6.0m
    valid = (Distances > 0.15) & (Distances < 6.0);
    
    front_mask = valid & (angles > 45*pi/180) & (angles < 135*pi/180);       % ด้านหน้า -30 ถึง +30 องศา
    left_mask  = valid & (angles < 45*pi/180) & (angles > -45*pi/180);     % ด้านซ้าย +30 ถึง +90 องศา
    right_mask = valid & (angles > 135*pi/180) & (angles < 225*pi/180);   % ด้านขวา -90 ถึง -30 องศา
    
    if any(front_mask)
        min_front = min(Distances(front_mask));
    else
        min_front = 999.0;
    end
    
    if any(left_mask)
        min_left = min(Distances(left_mask));
    else
        min_left = 999.0;
    end
    
    if any(right_mask)
        min_right = min(Distances(right_mask));
    else
        min_right = 999.0;
    end
end
